simulink model "boost_voltage_armature_control"  (R2016a)
settings: Solver=VariableStepAuto  StartTime=0.0  StopTime=0.6  RelTol=1e-3
libraries: powerlib x10, simulink x3, powerlib_meascontrol x1
settings Model: Creator=hi  LastModifiedBy=hi

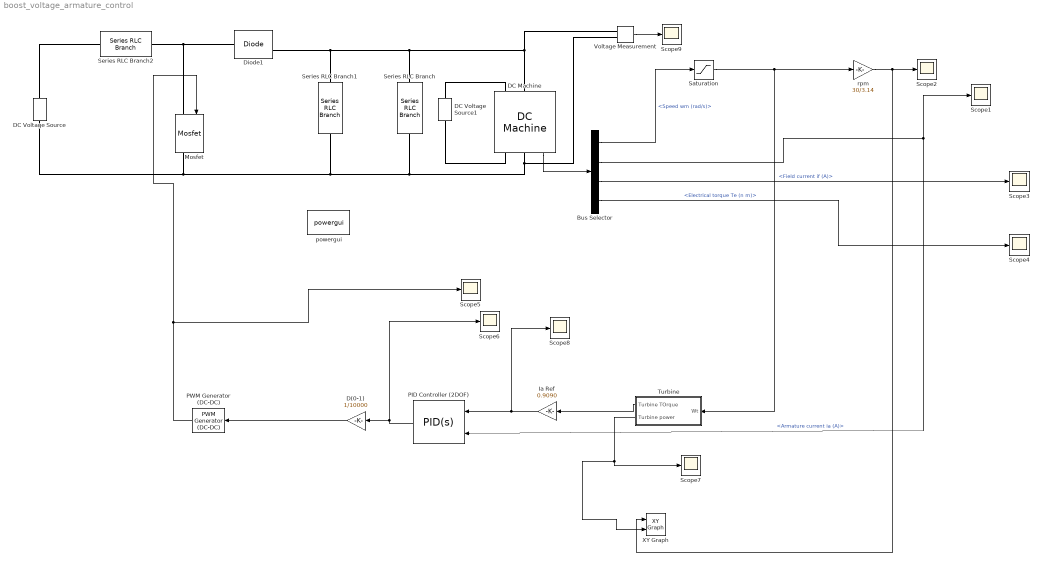
== system boost_voltage_armature_control ==
  Bus Selector : BusSelector  OutputSignals=Speed wm (rad/s),Armature current ia (A),Field current if (A),Electrical torque Te (n m)
  D(0-1) : Gain  Gain=1/10000  OutMin=[0]  OutMax=[1]
  DC Machine : powerlib/Machines/DC Machine  PresetModel=No  MechanicalLoad=Torque TL  FieldType=Wound  ShowDetailedParameters=on  MeasurementBus=off  RLa="[ 0.6  0.012]"  RLf="[ 240  120]"  Laf=1.8  MachineConstant=Torque constant (N.m/A)  Ke=1.8  Kt=1.8  J=1  Bm=0  Tf=0  w0=0.03  Ifinit=1  TsPowergui=0  TsBlock=-1
  DC Voltage Source : powerlib/Electrical Sources/DC Voltage Source  Amplitude=20  Measurements=None
  DC Voltage Source1 : powerlib/Electrical Sources/DC Voltage Source  Amplitude=150  Measurements=None
  Diode1 : powerlib/Power Electronics/Diode  Ron=0.001  Lon=0  Vf=0.8  IC=0  UseSnubber=off  Rs=500  Cs=250e-9  Measurements=on
  Ia Ref : Gain  Gain=0.9090
  Mosfet : powerlib/Power Electronics/Mosfet  Ron=0.001  Lon=0  Rd=0.001  Vfd=0  IC=0  Rs=1e5  Cs=inf  Measurements=on
  PID Controller (2DOF) : simulink/Continuous/PID Controller (2DOF)  Controller=PID  TimeDomain=Continuous-time  SampleTime=-1  IntegratorMethod=Forward Euler  FilterMethod=Forward Euler  Form=Parallel  UseFilter=on  ControllerParametersSource=internal  P=1  I=0  D=0  N=100  b=1  c=1  InitialConditionSource=internal  InitialConditionForIntegrator=0  InitialConditionForFilter=0  ExternalReset=none  LimitOutput=off  UpperSaturationLimit=inf  LowerSaturationLimit=-inf  LinearizeAsGain=on  AntiWindupMode=none  Kb=1  TrackingMode=off  Kt=1  PParamMin=[]  PParamMax=[]  IParamMin=[]  IParamMax=[]  DParamMin=[]  DParamMax=[]  NParamMin=[]  NParamMax=[]  bParamMin=[]  bParamMax=[]  cParamMin=[]  cParamMax=[]  KbParamMin=[]  KbParamMax=[]  KtParamMin=[]  KtParamMax=[]  POutMin=[]  POutMax=[]  IOutMin=[]  IOutMax=[]  DOutMin=[]  DOutMax=[]  NOutMin=[]  NOutMax=[]  bOutMin=[]  bOutMax=[]  cOutMin=[]  cOutMax=[]  KbOutMin=[]  KbOutMax=[]  KtOutMin=[]  KtOutMax=[]  IntegratorOutMin=[]  IntegratorOutMax=[]  FilterOutMin=[]  FilterOutMax=[]  SumOutMin=[]  SumOutMax=[]  Sum1OutMin=[]  Sum1OutMax=[]  Sum2OutMin=[]  Sum2OutMax=[]  Sum3OutMin=[]  Sum3OutMax=[]  SumI1OutMin=[]  SumI1OutMax=[]  SumI2OutMin=[]  SumI2OutMax=[]  SumI3OutMin=[]  SumI3OutMax=[]  SumDOutMin=[]  SumDOutMax=[]  SaturationOutMin=[]  SaturationOutMax=[]  IntegratorContinuousStateAttributes=''  IntegratorStateMustResolveToSignalObject=off  IntegratorRTWStateStorageClass=Auto  FilterContinuousStateAttributes=''  FilterStateMustResolveToSignalObject=off  FilterRTWStateStorageClass=Auto  DifferentiatorICPrevScaledInput=0  DifferentiatorOutMin=[]  DifferentiatorOutMax=[]
  PWM Generator (DC-DC) : powerlib_meascontrol/Pulse & Signal Generators/PWM Generator (DC-DC)  Fsw=5000  Ts=0
  Saturation : Saturate  UpperLimit=8.936066666666932  LowerLimit=0  OutMin=0  OutMax=8.936066666666932
  Scope{1..9} (9 alike) : Scope
  Series RLC Branch : powerlib/Elements/Series RLC Branch  LConnTagsString=__new0  RConnTagsString=__new0  BranchType=R  Resistance=100  Inductance=1e-3  SetiL0=off  InitialCurrent=0  Capacitance=1e-6  Setx0=off  InitialVoltage=0  Measurements=None
  Series RLC Branch1 : powerlib/Elements/Series RLC Branch  LConnTagsString=__new0  RConnTagsString=__new0  BranchType=C  Resistance=1  Inductance=1e-3  SetiL0=off  InitialCurrent=0  Capacitance=33e-6  Setx0=off  InitialVoltage=0  Measurements=None
  Series RLC Branch2 : powerlib/Elements/Series RLC Branch  LConnTagsString=__new0  RConnTagsString=__new0  BranchType=L  Resistance=1  Inductance=1e-3  SetiL0=off  InitialCurrent=0  Capacitance=1e-6  Setx0=off  InitialVoltage=0  Measurements=None
  "Turbine " : Subsystem
  Voltage Measurement : powerlib/Measurements/Voltage Measurement  PhasorSimulation=off  OutputType=Complex  PSBequivalent=0
  XY Graph : simulink/Sinks/XY Graph  xmin=0  xmax=90  ymin=0  ymax=70000  st=-1
  powergui : powerlib/powergui  Priority=1  SimulationMode=Continuous  SolverType=Tustin/Backward Euler (TBE)  SampleTime=50e-6  frequency=60  SPID=off  DisableSnubberDevices=off  DisableRonSwitches=off  DisableVfSwitches=off  SwTol=0  DisplayEquations=off  Interpol=off  ExternalGateDelay=off  methode=off  Ts=10  FunctionMessages=off  echomessages=off  HookPort=off  EnableUseOfTLC=off  x0status=zero  frequencyindice=0  Pbase=100e6  ErrMax=1e-4  Iterations=50  UnitsV=kV  UnitsW=MW  buscounter=0  RestoreLinks=warning  ResistiveCurrentMeasurement=off  Frange=[0:2:500]  Ylog=off  Xlog=on  ShowGrid=off  save=off  variable=ZData  structure=0  ZoomFFT=off  StartTime=0.0  cycles=1  DisplayStyle=1  fundamental=60  FreqAxis=off  MaxFrequency=1000  frequencyindicesteady=1  RmsSteady=1  display=off
  rpm : Gain  Gain=30/3.14
  wires:
  DC Machine/1 -> Bus Selector/1
  Bus Selector/1 -> Saturation/1  "<Speed wm (rad/s)>"
  Bus Selector/2 -> Scope1/1, PID Controller (2DOF)/2  "<Armature current ia (A)>"
  Bus Selector/3 -> Scope3/1  "<Field current if (A)>"
  Bus Selector/4 -> Scope4/1  "<Electrical torque Te (n m)>"
  rpm/1 -> XY Graph/1, Scope2/1
  "Turbine "/1(Turbine TOrque) -> Ia Ref/1
  Ia Ref/1 -> Scope8/1, PID Controller (2DOF)/1
  PID Controller (2DOF)/1 -> Scope6/1, D(0-1)/1
  PWM Generator (DC-DC)/1 -> Mosfet/1, Scope5/1
  D(0-1)/1 -> PWM Generator (DC-DC)/1
  "Turbine "/2(Turbine power) -> XY Graph/2, Scope7/1
  Voltage Measurement/1 -> Scope9/1
  Saturation/1 -> "Turbine "/1(Wt), rpm/1
  connections:
  Diode1/LConn1 -- Series RLC Branch2/RConn1 -- Mosfet/LConn1
  DC Voltage Source/LConn1 -- Mosfet/RConn1 -- Series RLC Branch1/RConn1 -- Series RLC Branch/RConn1 -- Voltage Measurement/LConn2 -- DC Machine/RConn1
  Series RLC Branch1/LConn1 -- Diode1/RConn1 -- DC Machine/LConn1 -- Voltage Measurement/LConn1 -- Series RLC Branch/LConn1
  DC Voltage Source/RConn1 -- Series RLC Branch2/LConn1
  DC Voltage Source1/RConn1 -- DC Machine/LConn2
  DC Voltage Source1/LConn1 -- DC Machine/RConn2

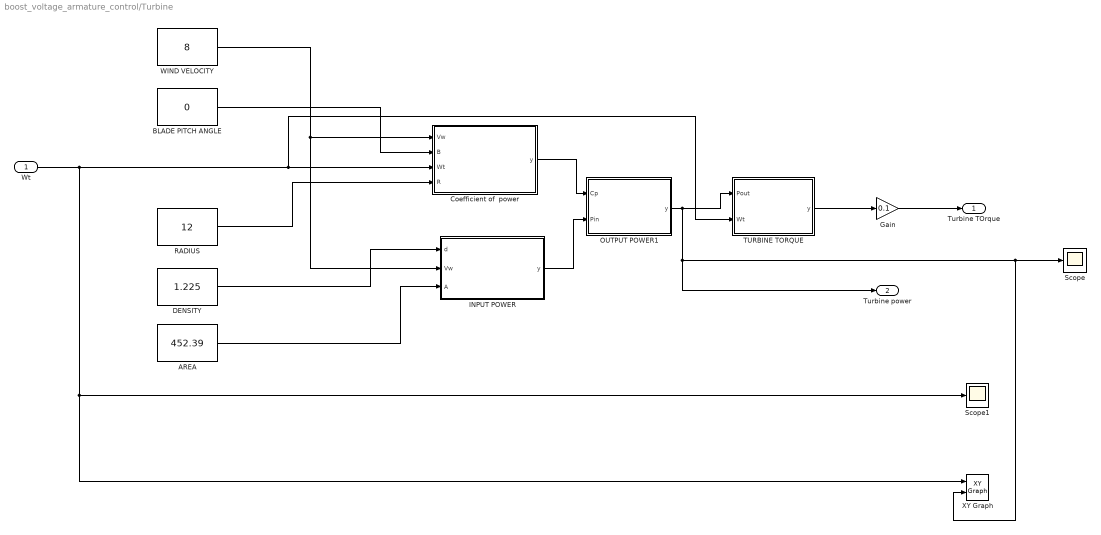
== system boost_voltage_armature_control/Turbine  ==
  Wt : Inport
  AREA : Constant  Value=452.39
  BLADE PITCH ANGLE : Constant  Value=0
  Coefficient of  power : MATLAB Function  TreatAsAtomicUnit=on
  DENSITY : Constant  Value=1.225
  Gain : Gain  Gain=0.1
  INPUT POWER : MATLAB Function  TreatAsAtomicUnit=on
  OUTPUT POWER1 : MATLAB Function  TreatAsAtomicUnit=on
  RADIUS : Constant  Value=12
  Scope : Scope
  Scope1 : Scope
  TURBINE TORQUE : MATLAB Function  TreatAsAtomicUnit=on
  WIND VELOCITY : Constant  Value=8
  XY Graph : simulink/Sinks/XY Graph  xmin=0  xmax=10  ymin=0  ymax=70000  st=-1
  Turbine TOrque : Outport
  Turbine power : Outport  Port=2
  wires:
  RADIUS/1 -> Coefficient of  power/4(R)
  BLADE PITCH ANGLE/1 -> Coefficient of  power/2(B)
  WIND VELOCITY/1 -> INPUT POWER/2(Vw), Coefficient of  power/1(Vw)
  DENSITY/1 -> INPUT POWER/1(d)
  AREA/1 -> INPUT POWER/3(A)
  INPUT POWER/1(y) -> OUTPUT POWER1/2(Pin)
  Coefficient of  power/1(y) -> OUTPUT POWER1/1(Cp)
  OUTPUT POWER1/1(y) -> Turbine power/1, XY Graph/2, Scope/1, TURBINE TORQUE/1(Pout)
  TURBINE TORQUE/1(y) -> Gain/1
  Gain/1 -> Turbine TOrque/1
  Wt/1 -> XY Graph/1, Scope1/1, TURBINE TORQUE/2(Wt), Coefficient of  power/3(Wt)

== matlab function boost_voltage_armature_control/Turbine /OUTPUT POWER1 ==
  data: Cp input; y output; Pin input
function y = fcn(Cp,Pin)
%#codegen

y = Cp*Pin;

== matlab function boost_voltage_armature_control/Turbine /INPUT POWER ==
  data: d input; y output; Vw input; A input
function y = fcn(d,Vw,A)
%#codegen

y = 0.5*d*Vw*Vw*Vw*A;

== matlab function boost_voltage_armature_control/Turbine /TURBINE TORQUE ==
  data: Pout input; y output; Wt input
function y = fcn(Pout,Wt)
%#codegen

y = Pout/Wt;

== matlab function boost_voltage_armature_control/Turbine /Coefficient of  power ==
  data: Vw input; y output; B input; Wt input; R input
function y = fcn(Vw,B,Wt,R)
%#codegen
lambda=(Wt*R)/Vw;
ki= (1/(lambda+0.08*B))-(0.035/(B*B*B+1));
y =( 0.5176*(116*ki-0.4*B-5)*exp(-21*ki))+(0.0068*lambda);
